simulink model "model_open_loop_integrator_regulator"  (Simulink 7.1)
settings: Solver=ode45  StartTime=0.0  StopTime=1000  RelTol=1e-3
undefined symbols (not defined in the file or in its folder): Ki, P
settings Model: Creator=ahp  LastModifiedBy=ahp

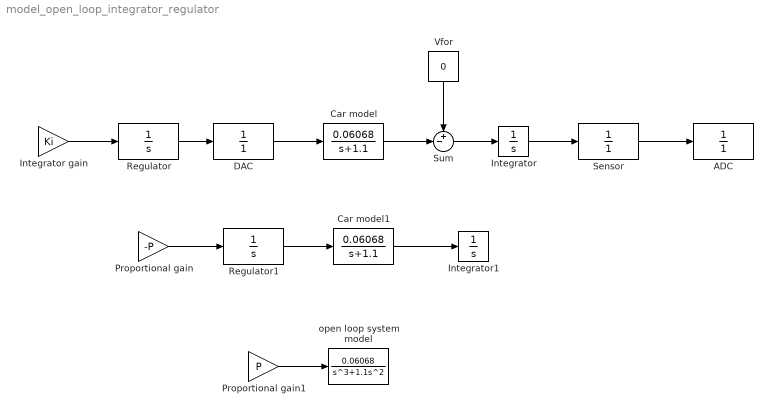
== system model_open_loop_integrator_regulator ==
  ADC : TransferFcn  Denominator=[1]
  Car model : TransferFcn  Numerator=[0.06068]  Denominator=[1 1.1]
  Car model1 : TransferFcn  Numerator=[0.06068]  Denominator=[1 1.1]
  DAC : TransferFcn  Denominator=[1]
  Integrator : Integrator
  Integrator gain : Gain  Gain=Ki  ParameterDataType=sfix(16)  ParameterScaling=2^0  OutDataType=sfix(16)  OutScaling=2^0
  Integrator1 : Integrator
  Proportional gain : Gain  Gain=-P  ParameterDataType=sfix(16)  ParameterScaling=2^0  OutDataType=sfix(16)  OutScaling=2^0
  Proportional gain1 : Gain  Gain=P  ParameterDataType=sfix(16)  ParameterScaling=2^0  OutDataType=sfix(16)  OutScaling=2^0
  Regulator : TransferFcn  Denominator=[1 0]
  Regulator1 : TransferFcn  Denominator=[1 0]
  Sensor : TransferFcn  Denominator=[1]
  Sum : Sum  Inputs=+-|  OutDataType=sfix(16)  OutScaling=2^0
  Vfor : Constant  Orientation=down  Value=0  OutDataType=sfix(16)  OutScaling=2^0
  open loop system model : TransferFcn  Numerator=[0.06068]  Denominator=[1 1.1 0 0]
  wires:
  Car model/1 -> Sum/2
  Regulator/1 -> DAC/1
  DAC/1 -> Car model/1
  Integrator/1 -> Sensor/1
  Sensor/1 -> ADC/1
  Integrator gain/1 -> Regulator/1
  Vfor/1 -> Sum/1
  Sum/1 -> Integrator/1
  Regulator1/1 -> Car model1/1
  Proportional gain/1 -> Regulator1/1
  Car model1/1 -> Integrator1/1
  Proportional gain1/1 -> open loop system model/1
